simulink subsystem "controls"  (R2025b)
settings: Solver=VariableStepAuto  StartTime=0.0  StopTime=10.0  RelTol=1e-3
undefined symbols (not defined in the file or in its folder): kappa_update_matlab, kappas, omegas, v_x
libraries: slpidlib x1
settings Model: Creator=jessi  LastModifiedBy=jessi

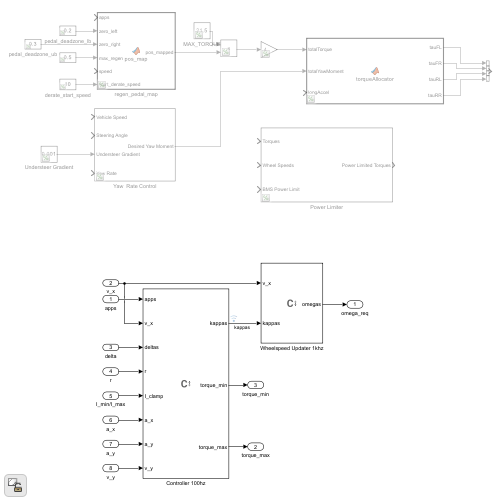
[thumbnail: Simulink's stored preview of the top-level diagram]
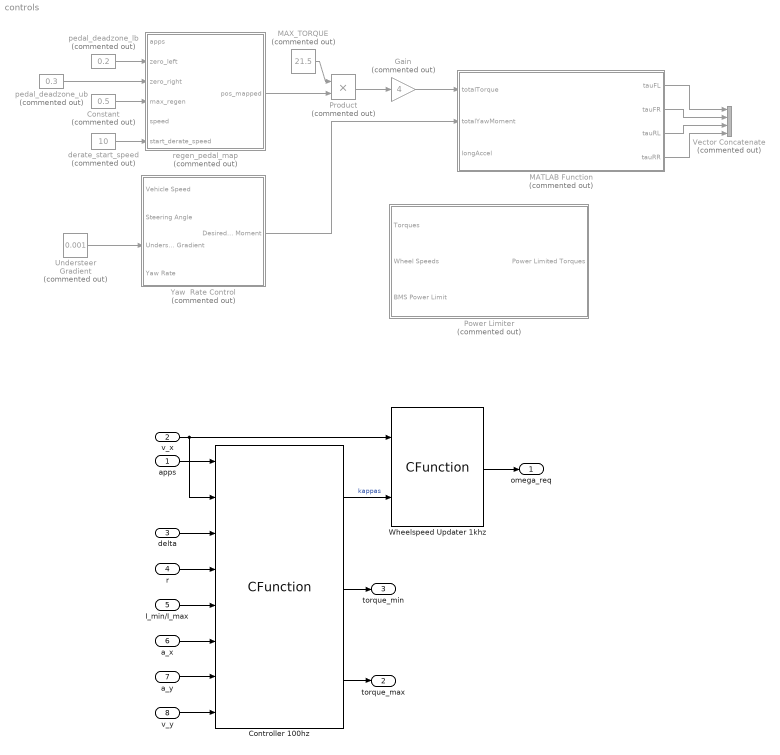
== system controls ==
  apps : Inport  Unit=%  PortDimensions=1
  v_x : Inport  Port=2  Unit=m/s  PortDimensions=1
  delta : Inport  Port=3  Unit=rad  PortDimensions=2
  r : Inport  Port=4  Unit=rad/s  PortDimensions=1
  I_min/I_max : Inport  Port=5  Unit=A  PortDimensions=1
  a_x : Inport  Port=6  Unit=m/s^2  PortDimensions=1
  a_y : Inport  Port=7  Unit=m/s^2  PortDimensions=1
  v_y : Inport  Port=8  Unit=m/s  PortDimensions=1
  Constant : Constant  Commented=on  Value=0.5
  Controller 100hz : CFunction  OutputCode=|  CodegenOutputCode=|  SampleTime=1/100  SimCustomHeaderFile=C:\Users\jessi\Documents\School\fsae\Consolidated-Firmware\firmware\hexray\VC\src\app\torque_vectoring\torque_vectoring_matlab.h  SimCustomLibraries=C:\Users\jessi\Documents\School\fsae\Consolidated-Firmware\build_fw_test\firmware\hexray\VC\hexray_VC_torque_vectoring.lib  SimCustomSearchDirectory=|  CustomHeaderFile=C:\Users\jessi\Documents\School\fsae\Consolidated-Firmware\firmware\hexray\VC\src\app\torque_vectoring\torque_vectoring_matlab.h  CustomLibraries=C:\Users\jessi\Documents\School\fsae\Consolidated-Firmware\build_fw_test\firmware\hexray\VC\hexray_VC_torque_vectoring.lib  CustomSearchDirectory=|  SimCustomDefines=MATLAB  SimCustomCompilerFlags=/std:c++20  CustomDefines=MATLAB  CustomCompilerFlags=/std:c++20
      OutputCode=|
      | update_matlab(
      |     v_x, v_y, r, a_x, a_y, apps, deltas[0], deltas[1], kappas,
      |     torque_max,
      |     torque_min
      | );
      CodegenOutputCode=|
      | update_matlab(
      |     v_x, v_y, r, a_x, a_y, apps, deltas[0], deltas[1], kappas,
      |     torque_max,
      |     torque_min
      | );
      SimCustomSearchDirectory=|
      | C:\Users\jessi\Documents\School\fsae\Consolidated-Firmware\firmware\shared\srcpp\app
      | C:\Users\jessi\Documents\School\fsae\Consolidated-Firmware\firmware\shared\srcpp\util
      | C:\Users\jessi\Documents\School\fsae\Consolidated-Firmware\firmware\hexray\VC\src\app
      CustomSearchDirectory=|
      | C:\Users\jessi\Documents\School\fsae\Consolidated-Firmware\firmware\shared\srcpp\app
      | C:\Users\jessi\Documents\School\fsae\Consolidated-Firmware\firmware\shared\srcpp\util
      | C:\Users\jessi\Documents\School\fsae\Consolidated-Firmware\firmware\hexray\VC\src\app
  Gain : Gain  Commented=on  Gain=4
  MATLAB Function : MATLAB Function  Commented=on  TreatAsAtomicUnit=on
  MAX_TORQUE : Constant  Commented=on  Value=21.5
  Power Limiter : Subsystem  Commented=on
  Product : Product  Commented=on
  Understeer Gradient : Constant  Commented=on  Value=0.001
  Vector Concatenate : Concatenate  Commented=on  NumInputs=4
  Wheelspeed Updater 1khz : CFunction  OutputCode=kappa_update_matlab(kappas, v_x, omegas);  CodegenOutputCode=kappa_update_matlab(kappas, v_x, omegas);  SampleTime=1/1000  SimCustomHeaderFile=C:\Users\jessi\Documents\School\fsae\Consolidated-Firmware\firmware\hexray\VC\src\app\torque_vectoring\torque_vectoring_matlab.h  SimCustomSearchDirectory=|  CustomHeaderFile=C:\Users\jessi\Documents\School\fsae\Consolidated-Firmware\firmware\hexray\VC\src\app\torque_vectoring\torque_vectoring_matlab.h  CustomSearchDirectory=|  SimCustomCompilerFlags=/std:c++20  CustomCompilerFlags=/std:c++20
      SimCustomSearchDirectory=|
      | C:\Users\jessi\Documents\School\fsae\Consolidated-Firmware\firmware\shared\srcpp\app
      | C:\Users\jessi\Documents\School\fsae\Consolidated-Firmware\firmware\shared\srcpp\util
      | C:\Users\jessi\Documents\School\fsae\Consolidated-Firmware\firmware\hexray\VC\src\app
      | C:\Users\jessi\Documents\School\fsae\Consolidated-Firmware\build_fw_dev\_deps\eigen-src
      | C:\Users\jessi\Documents\School\fsae\Consolidated-Firmware\build_fw_dev\_deps\auto_diff-src
      | C:\Users\jessi\Documents\School\fsae\Consolidated-Firmware\build_fw_dev\_deps\auto_diff-src\autodiff\forward
      | C:\Users\jessi\Documents\School\fsae\Consolidated-Firmware\build_fw_dev\_deps\auto_diff-src\autodiff\forward\utils
      CustomSearchDirectory=|
      | C:\Users\jessi\Documents\School\fsae\Consolidated-Firmware\firmware\shared\srcpp\app
      | C:\Users\jessi\Documents\School\fsae\Consolidated-Firmware\firmware\shared\srcpp\util
      | C:\Users\jessi\Documents\School\fsae\Consolidated-Firmware\firmware\hexray\VC\src\app
      | C:\Users\jessi\Documents\School\fsae\Consolidated-Firmware\build_fw_dev\_deps\eigen-src
      | C:\Users\jessi\Documents\School\fsae\Consolidated-Firmware\build_fw_dev\_deps\auto_diff-src
      | C:\Users\jessi\Documents\School\fsae\Consolidated-Firmware\build_fw_dev\_deps\auto_diff-src\autodiff\forward
      | C:\Users\jessi\Documents\School\fsae\Consolidated-Firmware\build_fw_dev\_deps\auto_diff-src\autodiff\forward\utils
  Yaw  Rate Control : Subsystem  Commented=on
  derate_start_speed : Constant  Commented=on  Value=10
  pedal_deadzone_lb : Constant  Commented=on  Value=0.2
  pedal_deadzone_ub : Constant  Commented=on  Value=0.3
  regen_pedal_map : MATLAB Function  Commented=on  TreatAsAtomicUnit=on
  omega_req : Outport  Unit=rad/s  PortDimensions=4
  torque_max : Outport  Port=2  Unit=N*m  PortDimensions=4
  torque_min : Outport  Port=3  Unit=N*m  PortDimensions=4
  wires:
  MAX_TORQUE/1 -> Product/1
  regen_pedal_map/1(pos_mapped) -> Product/2
  pedal_deadzone_lb/1 -> regen_pedal_map/2(zero_left)
  pedal_deadzone_ub/1 -> regen_pedal_map/3(zero_right)
  Constant/1 -> regen_pedal_map/4(max_regen)
  derate_start_speed/1 -> regen_pedal_map/6(start_derate_speed)
  Product/1 -> Gain/1
  Understeer Gradient/1 -> Yaw  Rate Control/3(Understeer Gradient)
  MATLAB Function/1(tauFL) -> Vector Concatenate/1
  MATLAB Function/2(tauFR) -> Vector Concatenate/2
  MATLAB Function/3(tauRL) -> Vector Concatenate/3
  MATLAB Function/4(tauRR) -> Vector Concatenate/4
  Yaw  Rate Control/1(Desired Yaw Moment) -> MATLAB Function/2(totalYawMoment)
  Gain/1 -> MATLAB Function/1(totalTorque)
  apps/1 -> Controller 100hz/1
  v_x/1 -> Controller 100hz/2, Wheelspeed Updater 1khz/1
  delta/1 -> Controller 100hz/3
  r/1 -> Controller 100hz/4
  I_min/I_max/1 -> Controller 100hz/5
  a_x/1 -> Controller 100hz/6
  Controller 100hz/2 -> torque_min/1
  Wheelspeed Updater 1khz/1 -> omega_req/1
  a_y/1 -> Controller 100hz/7
  v_y/1 -> Controller 100hz/8
  Controller 100hz/3 -> torque_max/1
  Controller 100hz/1 -> Wheelspeed Updater 1khz/2  "kappas"

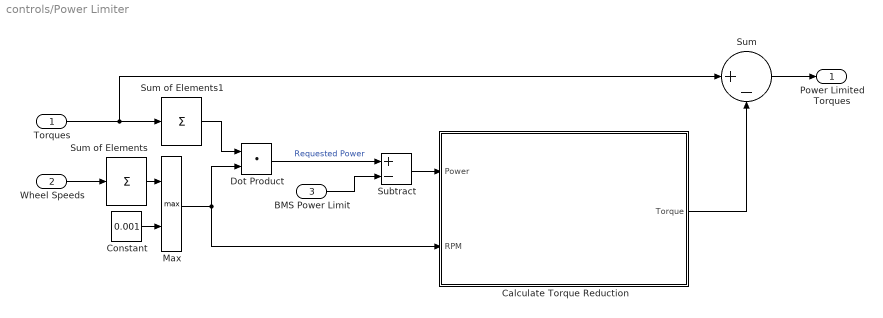
== system controls/Power Limiter ==
  Torques : Inport
  Wheel Speeds : Inport  Port=2
  BMS Power Limit : Inport  Port=3
  Calculate Torque Reduction : Subsystem
  Constant : Constant  Value=0.001
  Dot Product : DotProduct  OutDataTypeStr=Inherit: Inherit via internal rule
  Max : MinMax  Function=max  Inputs=2
  Subtract : Sum  Inputs=+-
  Sum : Sum  Inputs=|+-
  Sum of Elements : Sum  Inputs=+  CollapseDim=4
  Sum of Elements1 : Sum  Inputs=+  CollapseDim=4
  Power Limited Torques : Outport
  wires:
  Constant/1 -> Max/2
  Sum of Elements/1 -> Max/1
  Max/1 -> Dot Product/2, Calculate Torque Reduction/2(RPM)
  Sum/1 -> Power Limited Torques/1
  Calculate Torque Reduction/1(Torque) -> Sum/2
  Subtract/1 -> Calculate Torque Reduction/1(Power)
  Sum of Elements1/1 -> Dot Product/1
  BMS Power Limit/1 -> Subtract/2
  Dot Product/1 -> Subtract/1  "Requested Power"
  Wheel Speeds/1 -> Sum of Elements/1
  Torques/1 -> Sum/1, Sum of Elements1/1

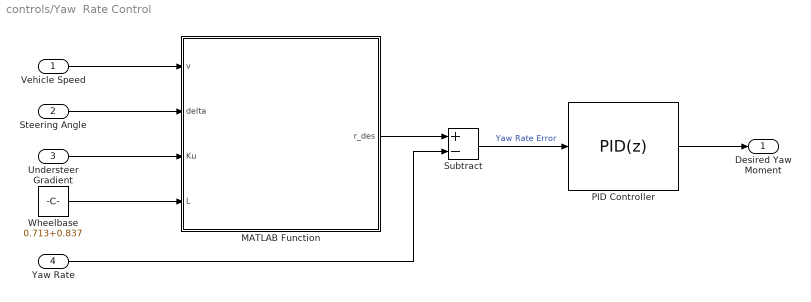
== system controls/Yaw  Rate Control ==
  Vehicle Speed : Inport
  Steering Angle : Inport  Port=2
  Understeer Gradient : Inport  Port=3
  Yaw Rate : Inport  Port=4
  MATLAB Function : MATLAB Function  TreatAsAtomicUnit=on
  PID Controller : slpidlib/PID Controller  Controller=PID  Form=Parallel  TimeDomain=Discrete-time  UseExternalTs=off  SampleTime=-1  IntegratorMethod=Forward Euler  FilterMethod=Forward Euler  ControllerParametersSource=internal  P=1  I=0  UseKiTs=off  D=0  UseExternalDerivativeSource=off  N=100  UseFilter=off  TunerSelectOption=Transfer Function Based (PID Tuner App)  InitialConditionSource=internal  InitialConditionForIntegrator=0  InitialConditionForFilter=0  DifferentiatorICPrevScaledInput=0  ExternalReset=none  TrackingMode=off  Kt=1  LimitOutput=off  SatLimitsSource=internal  UpperSaturationLimit=inf  LowerSaturationLimit=-inf  LinearizeAsGain=on  AntiWindupMode=none  Kb=1  LimitIntegrator=off  UpperIntegratorSaturationLimit=inf  LowerIntegratorSaturationLimit=-inf  POutMin=[]  POutMax=[]  IOutMin=[]  IOutMax=[]  DOutMin=[]  DOutMax=[]  NOutMin=[]  NOutMax=[]  SumOutMin=[]  SumOutMax=[]  SaturationOutMin=[]  SaturationOutMax=[]  PParamMin=[]  PParamMax=[]  IParamMin=[]  IParamMax=[]  DParamMin=[]  DParamMax=[]  NParamMin=[]  NParamMax=[]  KbParamMin=[]  KbParamMax=[]  KtParamMin=[]  KtParamMax=[]  KbOutMin=[]  KbOutMax=[]  KtOutMin=[]  KtOutMax=[]  IntegratorOutMin=[]  IntegratorOutMax=[]  FilterOutMin=[]  FilterOutMax=[]  SumI1OutMin=[]  SumI1OutMax=[]  SumI2OutMin=[]  SumI2OutMax=[]  SumI3OutMin=[]  SumI3OutMax=[]  SumI4OutMin=[]  SumI4OutMax=[]  SumDOutMin=[]  SumDOutMax=[]  DifferentiatorOutMin=[]  DifferentiatorOutMax=[]  FilterDiffOutCoefMin=[]  FilterDiffOutCoefMax=[]  ReciprocalOutMin=[]  ReciprocalOutMax=[]  SumDenOutMin=[]  SumDenOutMax=[]  SumNumOutMin=[]  SumNumOutMax=[]  DivideOutMin=[]  DivideOutMax=[]  UdiffTsProdOutMin=[]  UdiffTsProdOutMax=[]  NTsProdOutMin=[]  NTsProdOutMax=[]  UintegralTsProdOutMin=[]  UintegralTsProdOutMax=[]  UngainTsProdOutMin=[]  UngainTsProdOutMax=[]  ClampingZeroOutDataTypeStr=Inherit: Inherit via back propagation  ClampingZeroOutMin=[]  ClampingZeroOutMax=[]  FilterDenConstantOutDataTypeStr=Inherit: Inherit via back propagation  FilterDenConstantOutMin=[]  FilterDenConstantOutMax=[]  PCopyOutDataTypeStr=Inherit: Inherit via back propagation  PCopyOutMin=[]  PCopyOutMax=[]  NCopyOutDataTypeStr=Inherit: Inherit via back propagation  NCopyOutMin=[]  NCopyOutMax=[]  IntegratorContinuousStateAttributes=''  IntegratorStateMustResolveToSignalObject=off  IntegratorRTWStateStorageClass=Auto  FilterContinuousStateAttributes=''  FilterStateMustResolveToSignalObject=off  FilterRTWStateStorageClass=Auto  ParallelPVariant=InternalParameters  IdealPVariant=Disabled  IVariant=InternalParameters  DVariant=InternalParameters  IntegratorVariant=Discrete  SatVariant=Disabled  AWVariant=Passthrough  PCopyVariant=Disabled  TRVariant=Disabled  FdbkBlocksVariant=Forward  IdealPFdbkVariant=Disabled  SatFdbkVariant=Disabled  DerivativeFilterVariant=Differentiator  NVariant=Passthrough  NCopyVariant=Disabled_SignalSpec  FilterICVariant=InternalICsDifferentiator  IntegratorICVariant=InternalICs  ExternalResetVariant=Disabled  TRSumVariant=Passthrough  SumFdbkVariant=Disabled  SumVariant=Sum_PID  TsampFilterVariant=InternalTs  TsampNgainVariant=Passthrough  TsampIntegralVariant=Disabled_SignalSpec  ExternalSaturationOutDataTypeStr=Inherit: Same as second input  DerivativeSourceVariant=ErrorSignal  PreIntVariant=InternalPreInt
  Subtract : Sum  Inputs=+-
  Wheelbase : Constant  Value=0.713+0.837
  Desired Yaw Moment : Outport
  wires:
  Subtract/1 -> PID Controller/1  "Yaw Rate Error"
  MATLAB Function/1(r_des) -> Subtract/1
  PID Controller/1 -> Desired Yaw Moment/1
  Vehicle Speed/1 -> MATLAB Function/1(v)
  Wheelbase/1 -> MATLAB Function/4(L)
  Yaw Rate/1 -> Subtract/2
  Understeer Gradient/1 -> MATLAB Function/3(Ku)
  Steering Angle/1 -> MATLAB Function/2(delta)

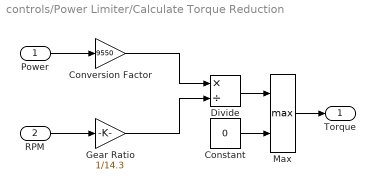
== system controls/Power Limiter/Calculate Torque Reduction ==
  Power : Inport
  RPM : Inport  Port=2
  Constant : Constant  Value=0
  Conversion Factor : Gain  Gain=9550
  Divide : Product  Inputs=*/
  Gear Ratio : Gain  Gain=1/14.3
  Max : MinMax  Function=max  Inputs=2
  Torque : Outport
  wires:
  Divide/1 -> Max/1
  RPM/1 -> Gear Ratio/1
  Max/1 -> Torque/1
  Constant/1 -> Max/2
  Gear Ratio/1 -> Divide/2
  Conversion Factor/1 -> Divide/1
  Power/1 -> Conversion Factor/1

== matlab function controls/MATLAB Function ==
  data: totalTorque input; tauFL output; totalYawMoment input; longAccel input; tauFR output; tauRL output; tauRR output
function [tauFL, tauFR, tauRL, tauRR] = ...
    torqueAllocator(totalTorque, totalYawMoment, longAccel)
%#codegen
% Inputs:
%   totalTorque    : total drive torque request [N·m]
%   totalYawMoment : desired total yaw moment about CG [N·m]
%   longAccel      : longitudinal acceleration (vehicle CG) [m/s^2]
%
% Outputs:
%   tauFL, tauFR, tauRL, tauRR : wheel torques [N·m] for [FL, FR, RL, RR]
%   loadTransferConst          : scalar per your Kmz formula
%   Mf, Mr                     : front/rear yaw-moment portions
%   F                          : axle moment-to-torque gain (SI-consistent)

% ===== Vehicle constants (edit to match your car) =====
g               = 9.80665;      % standard gravity [m/s^2] (exact by definition). 
wheelbase_m     = 1.55;         % given
mass_kg         = 300;          % vehicle + driver (adjust if needed)
cgHeight_m      = 0.30;         % CG height
distFrontAxleCG = 0.837;        % distance from front axle to CG
track_m         = 1.10;         % track width
wheel_diam_in   = 18;           % wheel/tire diameter (inches)
gear_ratio      = 14.3;         % total ratio to wheel torque

% ===== Compute F in meters (track / wheel_radius) * gear_ratio =====
wheel_radius_m  = (wheel_diam_in * 0.0254) / 2;
F = (track_m / wheel_radius_m) * gear_ratio;   % dimensionless gain

% ===== Load-transfer constant (Kmz) per your macros =====
% WEIGHT_ACROSS_BODY = (m*g)/wheelbase
W_ab = (mass_kg * g) / wheelbase_m;

% ACCELERATION_TERM_KMZ(a) = distFrontAxleCG + a*cgHeight/g
accTerm = distFrontAxleCG + (longAccel .* cgHeight_m ./ g);

% load_transfer_const =
%   ((m*g) - (W_ab * accTerm)) / (W_ab * accTerm)
loadTransferConst = ((mass_kg * g) - (W_ab .* accTerm)) ./ (W_ab .* accTerm);

% ===== Split total yaw moment between axles (your rule) =====
Mr = totalYawMoment ./ (1 + loadTransferConst);
Mf = totalYawMoment - Mr;

% ===== Base longitudinal split (per your formula) =====
front_base = (totalTorque .* loadTransferConst) ./ (2 .* (loadTransferConst + 1));
rear_base  = (totalTorque ./ 2) ...
           - (totalTorque .* loadTransferConst) ./ (2 .* (loadTransferConst + 1));

% ===== Apply axle yaw moments symmetrically across wheels =====
tauFL = front_base - (Mf ./ (2 .* F));
tauFR = front_base + (Mf ./ (2 .* F));

tauRL = rear_base  - (Mr ./ (2 .* F));   % includes rear yaw contribution
tauRR = rear_base  + (Mr ./ (2 .* F));
end

== matlab function controls/Yaw  Rate Control/MATLAB Function ==
  data: v input; r_des output; delta input; Ku input; L input
function r_des = desired_yaw_rate(v, delta, Ku, L)

r_des = (v * delta) / (L + (Ku * (v ^ 2)));

== matlab function controls/regen_pedal_map ==
  data: apps input; pos_mapped output; zero_left input; zero_right input; max_regen input; speed input; start_derate_speed input
function pos_mapped = pos_map(apps, zero_left, zero_right, max_regen, speed, start_derate_speed)
    if apps < zero_left
        % regen condition
        unclipped_derate_term = (speed - 5)/(start_derate_speed - 5);
        derate_term = max(0, min(1, unclipped_derate_term));
        pos_mapped = (apps - zero_left) / zero_left * max_regen * derate_term;
    elseif zero_left <= apps && apps <= zero_right
        pos_mapped = 0;
    else % apps > zero_right
        pos_mapped = (apps-zero_right)/(1-zero_right);
    end
end
